simulink model "q1"  (R2024a)
settings: Solver=VariableStepAuto  StartTime=0.0  StopTime=15  MaxStep=1e-4  RelTol=1e-3
settings Model: Creator=SHINE MOHAN S  LastModifiedBy=SHINE MOHAN S

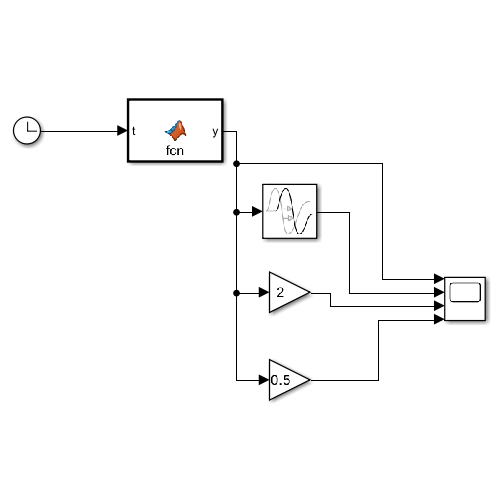
[thumbnail: Simulink's stored preview of the top-level diagram]
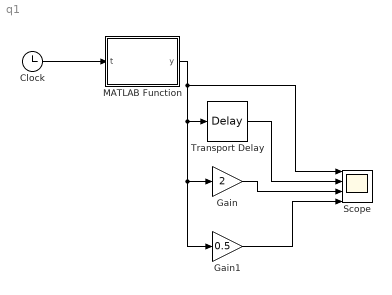
== system q1 ==
  Clock : Clock
  Gain : Gain  Gain=2
  Gain1 : Gain  Gain=0.5
  MATLAB Function : MATLAB Function  TreatAsAtomicUnit=on
  Scope : Scope  NumInputPorts=4
  Transport Delay : TransportDelay  DelayTime=3
  wires:
  Clock/1 -> MATLAB Function/1(t)
  MATLAB Function/1(y) -> Scope/1, Gain1/1, Gain/1, Transport Delay/1
  Transport Delay/1 -> Scope/2
  Gain/1 -> Scope/3
  Gain1/1 -> Scope/4

== matlab function q1/MATLAB Function ==
  data: t input; y output
function y = fcn(t)
    if t >= 0 && t < 2
        y = t;
    elseif t >= 2 && t <= 6
        y = 2;
    elseif t > 6 && t <= 8
        y = 8 - t;
    else
        y = 0;
    end
end
